simulink model "example21and22"  (R2023b)
settings: Solver=VariableStepAuto  StartTime=0.0  StopTime=10.0  RelTol=1e-3
settings Model: Creator=ray  LastModifiedBy=ray

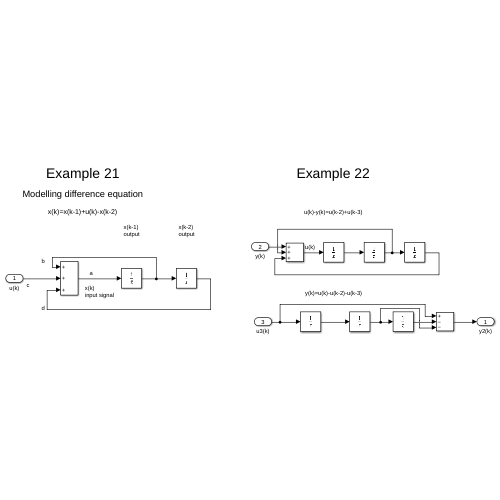
[thumbnail: Simulink's stored preview of the top-level diagram]
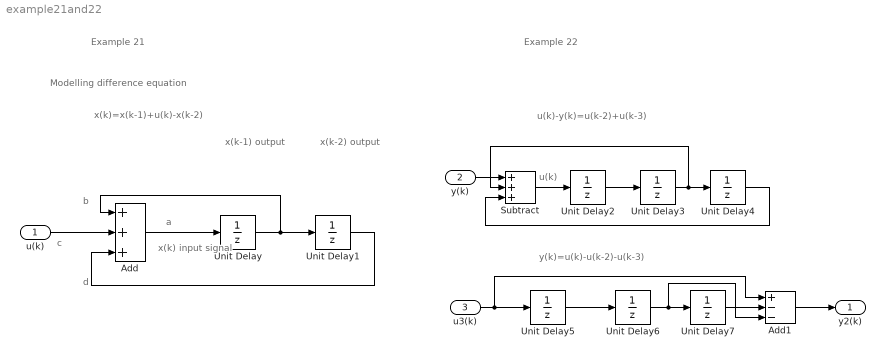
== system example21and22 ==
  note: y(k)=u(k)-u(k-2)-u(k-3)
  note: u(k)
  note: Example 22
  note: u(k)-y(k)=u(k-2)+u(k-3)
  note: d
  note: c
  note: b
  note: a
  note: x(k-2)
      | output
  note: x(k-1)
      | output
  note: x(k)
      | input signal
  note: x(k)=x(k-1)+u(k)-x(k-2)
  note: Modelling difference equation
  note: Example 21
  u(k) : Inport
  y(k) : Inport  Port=2
  u3(k) : Inport  Port=3
  Add : Sum  Inputs=+++
  Add1 : Sum  Inputs=+--
  Subtract : Sum  Inputs=+++
  Unit Delay{,1..7} (8 alike) : UnitDelay  SampleTime=-1  HasFrameUpgradeWarning=on
  y2(k) : Outport
  wires:
  Unit Delay/1 -> Add/1, Unit Delay1/1
  Add/1 -> Unit Delay/1
  Unit Delay1/1 -> Add/3
  u(k)/1 -> Add/2
  Unit Delay2/1 -> Unit Delay3/1
  Unit Delay3/1 -> Subtract/2, Unit Delay4/1
  y(k)/1 -> Subtract/1
  Subtract/1 -> Unit Delay2/1
  Unit Delay4/1 -> Subtract/3
  Add1/1 -> y2(k)/1
  Unit Delay7/1 -> Add1/2
  u3(k)/1 -> Add1/1, Unit Delay5/1
  Unit Delay5/1 -> Unit Delay6/1
  Unit Delay6/1 -> Add1/3, Unit Delay7/1
